simulink model "ZeroForceDrag_SingleJoint"  (R2018b)
settings: Solver=FixedStepDiscrete  StartTime=0.0  StopTime=Inf  FixedStep=0.001  RelTol=1e-3  EnableMultiTasking=on
undefined symbols (not defined in the file): J1, J2, J3, J4, J5, J6, J7, Motor_Current, Motor_Position, Motor_Velocity, Send_GUIdata
libraries: c280xlib x14, simulink x5, idelinklib_common x1
(part 1 of 4)
settings Model: ExtModeTrigDuration=8  Creator=Administrator  LastModifiedBy=Jeason
settings OptimizationCC: DefaultUnderspecifiedDataType=single  EnhancedBackFolding=on  PassReuseOutputArgsAs=Individual arguments  MaxStackSize=512  OptimizeBlockOrder=speed  DifferentSizesBufferReuse=on  OptimizationCustomize=off
settings DebuggingCC: InheritedTsInSrcMsg=none  MultiTaskDSMMsg=none  ParameterTunabilityLossMsg=error
settings HardwareCC: ProdBitPerChar=16  ProdBitPerInt=16  ProdBitPerPointer=32  ProdBitPerSizeT=32  ProdBitPerPtrDiffT=32  ProdLargestAtomicInteger=Integer  ProdLargestAtomicFloat=None  ProdWordSize=16  ProdLongLongMode=on  ProdHWDeviceType=Texas Instruments->C2000
settings SFSimCC: MATLABDynamicMemAlloc=off
settings RTWCC: SystemTargetFile=ert.tlc  HardwareBoard=TI Delfino F2833x  TemplateMakefile=ert_default_tmf  GenerateReport=on  Toolchain=Texas Instruments Code Composer Studio (C2000)  IncludeHyperlinkInReport=on  LaunchReport=on  GenerateTraceInfo=on  GenerateTraceReport=on  GenerateTraceReportSl=on  GenerateTraceReportSf=on  GenerateTraceReportEml=on
settings CodeAppCC: ForceParamTrailComments=on  IgnoreCustomStorageClasses=off  OperatorAnnotations=on  SimulinkDataObjDesc=on  SFDataObjDesc=on  InsertBlockDesc=on
settings ERTTargetCC: CodeReplacementLibrary=TI C28x

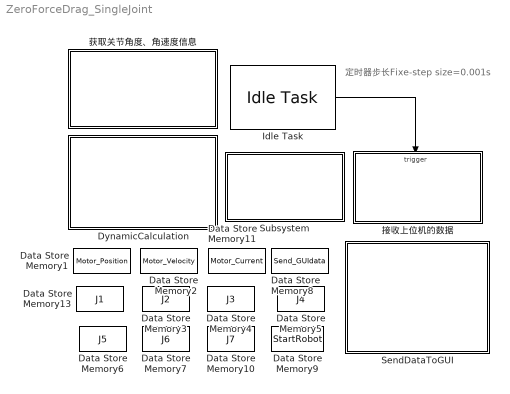
== system ZeroForceDrag_SingleJoint ==
  note: 定时器步长Fixe-step size=0.001s
  Data Store Memory1 : DataStoreMemory  DataStoreName=Motor_Position  ReadBeforeWriteMsg=warning  WriteAfterWriteMsg=warning  WriteAfterReadMsg=warning  InitialValue=[0 0 0 0 0 0]  ShowAdditionalParam=off  OutDataTypeStr=int32
      settings: RTWStateStorageClass=ExportedGlobal
  Data Store Memory10 : DataStoreMemory  DataStoreName=J7  ReadBeforeWriteMsg=warning  WriteAfterWriteMsg=warning  WriteAfterReadMsg=warning  InitialValue=[0 0 0 0 0 0]  ShowAdditionalParam=off  OutDataTypeStr=double
      settings: RTWStateStorageClass=ExportedGlobal
  Data Store Memory11 : DataStoreMemory  DataStoreName=Motor_Current  ReadBeforeWriteMsg=warning  WriteAfterWriteMsg=warning  WriteAfterReadMsg=warning  InitialValue=[0 0 0 0 0 0]  ShowAdditionalParam=off  OutDataTypeStr=int32
      settings: RTWStateStorageClass=ExportedGlobal
  Data Store Memory13 : DataStoreMemory  DataStoreName=J1  ReadBeforeWriteMsg=warning  WriteAfterWriteMsg=warning  WriteAfterReadMsg=warning  InitialValue=[0 0 0 0 0 0]  ShowAdditionalParam=off  OutDataTypeStr=double
      settings: RTWStateStorageClass=ExportedGlobal
  Data Store Memory2 : DataStoreMemory  DataStoreName=Motor_Velocity  ReadBeforeWriteMsg=warning  WriteAfterWriteMsg=warning  WriteAfterReadMsg=warning  InitialValue=[0 0 0 0 0 0]  ShowAdditionalParam=off  OutDataTypeStr=int32
      settings: RTWStateStorageClass=ExportedGlobal
  Data Store Memory3 : DataStoreMemory  DataStoreName=J2  ReadBeforeWriteMsg=warning  WriteAfterWriteMsg=warning  WriteAfterReadMsg=warning  InitialValue=[0 0 0 0 0 0]  ShowAdditionalParam=off  OutDataTypeStr=double
      settings: RTWStateStorageClass=ExportedGlobal
  Data Store Memory4 : DataStoreMemory  DataStoreName=J3  ReadBeforeWriteMsg=warning  WriteAfterWriteMsg=warning  WriteAfterReadMsg=warning  InitialValue=[0 0 0 0 0 0]  ShowAdditionalParam=off  OutDataTypeStr=double
      settings: RTWStateStorageClass=ExportedGlobal
  Data Store Memory5 : DataStoreMemory  DataStoreName=J4  ReadBeforeWriteMsg=warning  WriteAfterWriteMsg=warning  WriteAfterReadMsg=warning  InitialValue=[0 0 0 0 0 0]  ShowAdditionalParam=off  OutDataTypeStr=double
      settings: RTWStateStorageClass=ExportedGlobal
  Data Store Memory6 : DataStoreMemory  DataStoreName=J5  ReadBeforeWriteMsg=warning  WriteAfterWriteMsg=warning  WriteAfterReadMsg=warning  InitialValue=[0 0 0 0 0 0]  ShowAdditionalParam=off  OutDataTypeStr=double
      settings: RTWStateStorageClass=ExportedGlobal
  Data Store Memory7 : DataStoreMemory  DataStoreName=J6  ReadBeforeWriteMsg=warning  WriteAfterWriteMsg=warning  WriteAfterReadMsg=warning  InitialValue=[0 0 0 0 0 0]  ShowAdditionalParam=off  OutDataTypeStr=double
      settings: RTWStateStorageClass=ExportedGlobal
  Data Store Memory8 : DataStoreMemory  DataStoreName=Send_GUIdata  ReadBeforeWriteMsg=warning  WriteAfterWriteMsg=warning  WriteAfterReadMsg=warning  InitialValue=zeros(1,18)  ShowAdditionalParam=off  OutDataTypeStr=double
      settings: RTWStateStorageClass=ExportedGlobal
  Data Store Memory9 : DataStoreMemory  DataStoreName=StartRobot  ReadBeforeWriteMsg=warning  WriteAfterWriteMsg=warning  WriteAfterReadMsg=warning  ShowAdditionalParam=off  OutDataTypeStr=uint16
      settings: RTWStateStorageClass=ExportedGlobal
  DynamicCalculation : Subsystem  Tag=Calculated_Data  Priority=2  TreatAsAtomicUnit=on  RTWFcnName=DynamicsController
      settings: RTWSystemCode=Nonreusable function  RTWFcnNameOpts=User specified  RTWFileNameOpts=Use function name
      mask Display:
      | color('red')
      | disp('六轴机械臂\n单关节零力控制')
  Idle Task : idelinklib_common/Idle Task  tasknumbers=[0]  taskpriorities=100016  taskpreempts=[1]  showinput=off  simPriority=0
  SendDataToGUI : Subsystem  Priority=2  TreatAsAtomicUnit=on
      settings: RTWSystemCode=Nonreusable function
  Subsystem : Subsystem
      mask Display: disp('System\nInitialization');
  接收上位机的数据 : Subsystem  TreatAsAtomicUnit=on
  获取关节角度、角速度信息 : Subsystem  Tag=Get_Data  Priority=0  TreatAsAtomicUnit=on
      settings: RTWSystemCode=Nonreusable function
  wires:
  Idle Task/1 -> 接收上位机的数据/Trigger

== system ZeroForceDrag_SingleJoint/DynamicCalculation ==
  note: 转换为外转子的角度值
  note: 定义全局变量，各变量
      | 为[1x6]的矩阵
  note: 六轴机械臂单关节零力拖动
      | 默认关节2
  note: 在做实验时选择对应的关节电机
  note: 注：必须两人操作，一人扶着机械臂，另外一人负责操作软硬件。以下是简化版的步骤，具体细节以实验指导书为准。
      | 首先打开稳压电源开关给机械臂控制器供电，然后再打开机械臂电源开关,上电2~3s后，打开上位机，点击上位机示教界面的“ 启动 ”按钮，所有电机松开抱闸。
      | 上位机的“ 组号 ”输入 7 ，“ 数据1 ”输入 1 ，点击" 下发数据 "按钮，对应电机切换到力矩模式，然后用手托着机械臂，防止重力原因掉落。
      | 上位机的“ 组号 ”输入对应关节组号，“ 数据1~数据6 ”输入对应的数据，点击" 下发数据 "按钮，输出力矩值给电机。
      | 做完实验后，按下急停按钮，断开机械臂电源，机械臂切换到位置模式，处于锁死状态。（要想让机械臂所有关节回到零位置，需下载PTP程序）。
  Compensate : Subsystem  Priority=1  TreatAsAtomicUnit=on  RTWFcnName=Compensate
      settings: RTWSystemCode=Nonreusable function  RTWFcnNameOpts=User specified  RTWFileNameOpts=Use function name
  Data Store Write3 : DataStoreWrite  DataStoreName=Tau  DataStoreElements=Tau(1)#Tau(2)#Tau(3)#Tau(4)#Tau(5)#Tau(6)
  Demux : Demux  Outputs=6
  DriveMotor : Subsystem  TreatAsAtomicUnit=on  RTWFcnName=DrivrMotor  mask(DriverMotor){Motor1=off, Motor2=on, Motor3=off, Motor4=off, Motor5=off, Motor6=off}
      mask help:
      | 当其中一个Motor勾选时，表示将力矩输出给对应的电机；如果不勾选时，表示对应的电机不工作。
      | 比如：如果做单关节实验时，哪个电机要做实验就勾选对应的电机，其他电机一定要不勾选。
      | 关节1~3为CANB,关节4~6为CANA,驱动邮箱号为7~12。输入量的范围限定在-900~900。
      settings: RTWSystemCode=Nonreusable function  RTWFcnNameOpts=User specified  RTWFileNameOpts=Use function name
      mask Callback Motor1:
      | vssBlk1 = [gcb, '/BottomDriver/Joint1'];
      | choice1 = get_param(gcb,'Motor1');
      | if strcmp(choice1,'off')
      |         set_param(vssBlk1, 'Commented','on');
      |     else
      |         set_param(vssBlk1, 'Commented','off');
      | end
      | clear choice1 vssBlk1;
      mask Callback Motor2:
      | vssBlk2 = [gcb, '/BottomDriver/Joint2'];
      | choice2 = get_param(gcb,'Motor2');
      | if strcmp(choice2,'off')
      |         set_param(vssBlk2, 'Commented','on');
      |     else
      |         set_param(vssBlk2, 'Commented','off');
      | end
      | clear choice2 vssBlk2;
      mask Callback Motor3:
      | vssBlk3 = [gcb, '/BottomDriver/Joint3'];
      | choice3 = get_param(gcb,'Motor3');
      | if strcmp(choice3,'off')
      |         set_param(vssBlk3, 'Commented','on');
      |     else
      |         set_param(vssBlk3, 'Commented','off');
      | end
      | clear choice3 vssBlk3;
      mask Callback Motor4:
      | vssBlk4 = [gcb, '/BottomDriver/Joint4'];
      | choice4 = get_param(gcb,'Motor4');
      | if strcmp(choice4,'off')
      |         set_param(vssBlk4, 'Commented','on');
      |     else
      |         set_param(vssBlk4, 'Commented','off');
      | end
      | clear choice4 vssBlk4;
      mask Callback Motor5:
      | vssBlk5 = [gcb, '/BottomDriver/Joint5'];
      | choice5 = get_param(gcb,'Motor5');
      | if strcmp(choice5,'off')
      |         set_param(vssBlk5, 'Commented','on');
      |     else
      |         set_param(vssBlk5, 'Commented','off');
      | end
      | clear choice5 vssBlk5;
      mask Callback Motor6:
      | vssBlk6 = [gcb, '/BottomDriver/Joint6'];
      | choice6 = get_param(gcb,'Motor6');
      | if strcmp(choice6,'off')
      |         set_param(vssBlk6, 'Commented','on');
      |     else
      |         set_param(vssBlk6, 'Commented','off');
      | end
      | clear choice6 vssBlk6;
      mask Display:
      | disp('DriverMotor');
      | port_label('input', 1, 'Tau1');
      | port_label('input', 2, 'Tau2');
      | port_label('input', 3, 'Tau3');
      | port_label('input', 4, 'Tau4');
      | port_label('input', 5, 'Tau5');
      | port_label('input', 6, 'Tau6');
      | port_label('input', 7, 'Enable');
  Gain : Gain  Gain=180/pi
  GetAngleVelocity : Subsystem  Priority=0  TreatAsAtomicUnit=on  RTWFcnName=GetAngleVelocity
      settings: RTWSystemCode=Nonreusable function  RTWFcnNameOpts=User specified  RTWFileNameOpts=Use function name
  InitAngle : DataStoreRead  DataStoreName=InitAngle
  Tau1~6 : DataStoreRead  DataStoreName=Tau
  dq : DataStoreRead  DataStoreName=dq
  q : DataStoreRead  DataStoreName=q
  上位机监控窗口1~6——参数1 : DataStoreWrite  DataStoreName=Send_GUIdata  DataStoreElements=Send_GUIdata(1:6)
  上位机监控窗口1~6——参数2 : DataStoreWrite  DataStoreName=Send_GUIdata  DataStoreElements=Send_GUIdata(7:12)
  切换到电流模式 的使能信号 : DataStoreRead  DataStoreName=J7  DataStoreElements=J7(1)
  各个关节外转子采集 到的原始角度-初始角度 : DataStoreMemory  DataStoreName=q  ReadBeforeWriteMsg=warning  WriteAfterWriteMsg=warning  WriteAfterReadMsg=warning  InitialValue=zeros(1,6)  ShowAdditionalParam=off  OutDataTypeStr=double
      settings: RTWStateStorageClass=ExportedGlobal
  各个关节外转子采集 到的实际角速度 : DataStoreMemory  DataStoreName=dq  ReadBeforeWriteMsg=warning  WriteAfterWriteMsg=warning  WriteAfterReadMsg=warning  InitialValue=zeros(1,6)  ShowAdditionalParam=off  OutDataTypeStr=double
      settings: RTWStateStorageClass=ExportedGlobal
  各关节角度 : DataStoreWrite  DataStoreName=q
  各关节角速度 : DataStoreWrite  DataStoreName=dq
  给定各关节 初始角度 : DataStoreMemory  DataStoreName=InitAngle  ReadBeforeWriteMsg=warning  WriteAfterWriteMsg=warning  WriteAfterReadMsg=warning  InitialValue=zeros(1,6)  ShowAdditionalParam=off  OutDataTypeStr=double
      settings: RTWStateStorageClass=ExportedGlobal
  给定的各关节 初始角度 : DataStoreWrite  DataStoreName=InitAngle
  驱动各个关节 运动的力矩 : DataStoreMemory  DataStoreName=Tau  ReadBeforeWriteMsg=warning  WriteAfterWriteMsg=warning  WriteAfterReadMsg=warning  InitialValue=zeros(1,6)  ShowAdditionalParam=off  OutDataTypeStr=double
      settings: RTWStateStorageClass=ExportedGlobal
  wires:
  Demux/3 -> DriveMotor/3(Tau3)
  Demux/5 -> DriveMotor/5(Tau5)
  Demux/2 -> DriveMotor/2(Tau2)
  Tau1~6/1 -> 上位机监控窗口1~6——参数2/1, Demux/1
  Demux/4 -> DriveMotor/4(Tau4)
  切换到电流模式 的使能信号/1 -> DriveMotor/7(Enable)
  Demux/1 -> DriveMotor/1(Tau1)
  Demux/6 -> DriveMotor/6(Tau6)
  q/1 -> Gain/1, Compensate/1(q)
  dq/1 -> Compensate/3(dq)
  Compensate/1(Tau1) -> Data Store Write3/1
  Compensate/2(Tau2) -> Data Store Write3/2
  Compensate/3(Tau3) -> Data Store Write3/3
  Compensate/4(Tau4) -> Data Store Write3/4
  Compensate/5(Tau5) -> Data Store Write3/5
  Compensate/6(Tau6) -> Data Store Write3/6
  Gain/1 -> 上位机监控窗口1~6——参数1/1
  GetAngleVelocity/2(InitAngle(rad)) -> 给定的各关节 初始角度/1
  GetAngleVelocity/1(q(rad)) -> 各关节角度/1
  GetAngleVelocity/3(q_dot(rad/s)) -> 各关节角速度/1
  InitAngle/1 -> Compensate/2(InitAngle)

== system ZeroForceDrag_SingleJoint/SendDataToGUI ==
  note: Upper limit=9
  note: 发送数据给上位机
  note: 定时器步长Fixe-step size=0.001s,
      | 每10ms发送一次数据给上位机
  " " : Subsystem
  Constant : Constant  Value=true  OutDataTypeStr=boolean
  Constant1 : Constant  Value=false  OutDataTypeStr=boolean
  Switch : Switch  Criteria=u2 > Threshold
  广播周期 : simulink/Sources/Counter Limited  uplimit=9  tsamp=-1
  wires:
  Switch/1 -> " "/Enable
  广播周期/1 -> Switch/2
  Constant1/1 -> Switch/1
  Constant/1 -> Switch/3

== system ZeroForceDrag_SingleJoint/Subsystem ==
  Model Header : Subsystem  mask(Model Header){ShowInLibBrowser=0}
      mask prompts: ShowInLibBrowser "Simulink:masks:CustCodeMaskParam1_MP"
      settings: CopyFcn=cccopyfcn(gcb)  OpenFcn=ccopenfcn('Model Header')
      mask Help: eval('feval(''rtwprivate'',''rtwhelpview'',''rtw_model_header_block'')');
      mask Display: disp('Model\nHeader');
  Model Source : Subsystem  mask(Model Source){ShowInLibBrowser=0}
      mask prompts: ShowInLibBrowser "Simulink:masks:CustCodeMaskParam1_MP"
      settings: CopyFcn=cccopyfcn(gcb)  OpenFcn=ccopenfcn('Model Source')
      mask Help: eval('feval(''rtwprivate'',''rtwhelpview'',''rtw_model_source_block'')');
      mask Display: disp('Model\nSource');
  System Initialize : Subsystem  mask(System Initialize){ShowInLibBrowser=0}
      mask prompts: ShowInLibBrowser "Simulink:masks:CustCodeMaskParam1_MP"
      settings: CopyFcn=cccopyfcn(gcb)  OpenFcn=ccopenfcn('System Initialize Function')
      mask Help: eval('feval(''rtwprivate'',''rtwhelpview'',''rtw_sys_initialize_block'')');
      mask Display: disp('System\nInitialize');

== system ZeroForceDrag_SingleJoint/接收上位机的数据 ==
  note: 接收上位机数据
  function : TriggerPort  TriggerType=function-call  VariantControl=Variant
  0x0080 : simulink/Logic and Bit Operations/Compare To Constant  relop===  const=hex2dec('0080')  OutDataTypeStr=boolean
  0x88 : simulink/Logic and Bit Operations/Compare To Constant  relop===  const=hex2dec('0088')  OutDataTypeStr=boolean
  Compare To Constant1 : simulink/Logic and Bit Operations/Compare To Constant  relop===  const=hex2dec('0001')  OutDataTypeStr=boolean
  Compare To Constant2 : simulink/Logic and Bit Operations/Compare To Constant  relop===  const=hex2dec('0001')  OutDataTypeStr=boolean
  Data Store Read : DataStoreRead  DataStoreName=PTX
  Data Store Write2 : DataStoreWrite  DataStoreName=StartRobot
  Data Type Conversion : DataTypeConversion  OutDataTypeStr=int16
  Data Type Conversion3 : DataTypeConversion  OutDataTypeStr=double
  Data Type Conversion4 : DataTypeConversion  OutDataTypeStr=uint16
  Demux1 : Demux  Outputs=9
  Logical Operator : Logic  Inputs=4  AllPortsSameDT=off  OutDataTypeStr=boolean
  Mux1 : Mux  Inputs=6
  Subsystem : Subsystem
  Terminator3 : Terminator
  消息使能 : DataStoreMemory  DataStoreName=PTX  ReadBeforeWriteMsg=warning  WriteAfterWriteMsg=warning  WriteAfterReadMsg=warning  InitialValue=true  ShowAdditionalParam=off  OutDataTypeStr=boolean
  获取用户命令 : Subsystem  Priority=1  TreatAsAtomicUnit=on
      settings: RTWSystemCode=Nonreusable function
  wires:
  Compare To Constant2/1 -> Logical Operator/4
  Compare To Constant1/1 -> Logical Operator/3
  Data Store Read/1 -> Logical Operator/2
  Logical Operator/1 -> Data Type Conversion4/1
  0x0080/1 -> Logical Operator/1
  Demux1/4 -> Mux1/2, Compare To Constant2/1
  Demux1/3 -> Mux1/1, Compare To Constant1/1
  Demux1/1 -> 0x0080/1, 0x88/1
  获取用户命令/1(消息) -> Demux1/1
  Demux1/5 -> Mux1/3
  Demux1/6 -> Mux1/4
  Demux1/9 -> Terminator3/1
  Demux1/7 -> Mux1/5
  Demux1/8 -> Mux1/6
  Mux1/1 -> Data Type Conversion/1
  Data Type Conversion/1 -> Data Type Conversion3/1
  Data Type Conversion4/1 -> Data Store Write2/1
  Demux1/2 -> Subsystem/1(组号)
  Data Type Conversion3/1 -> Subsystem/2(数据)
  0x88/1 -> Subsystem/Enable

== system ZeroForceDrag_SingleJoint/获取关节角度、角速度信息 ==
  note: 获取关节电流、 角速度、 角度信息
  CANA_284_24 : Subsystem  Priority=4  TreatAsAtomicUnit=on
      settings: RTWSystemCode=Nonreusable function
      mask Display:
      | color('WHITE')
      | disp('JOINT4\n数据读取')
  CANA_285_25 : Subsystem  Priority=5  TreatAsAtomicUnit=on
      settings: RTWSystemCode=Nonreusable function
      mask Display:
      | color('WHITE')
      | disp('JOINT5\n数据读取')
  CANA_286_26 : Subsystem  Priority=6  TreatAsAtomicUnit=on
      settings: RTWSystemCode=Nonreusable function
      mask Display:
      | color('WHITE')
      | disp('JOINT6\n数据读取')
  CANB_281_21 : Subsystem  Priority=1  TreatAsAtomicUnit=on
      settings: RTWSystemCode=Nonreusable function
      mask Display:
      | color('WHITE')
      | disp('JOINT1\n数据读取')
  CANB_282_22 : Subsystem  Priority=2  TreatAsAtomicUnit=on
      settings: RTWSystemCode=Nonreusable function
      mask Display:
      | color('white')
      | disp('JOINT2\n数据读取')
  CANB_283_23 : Subsystem  Priority=3  TreatAsAtomicUnit=on
      settings: RTWSystemCode=Nonreusable function
      mask Display:
      | color('white')
      | disp('JOINT3\n数据读取')

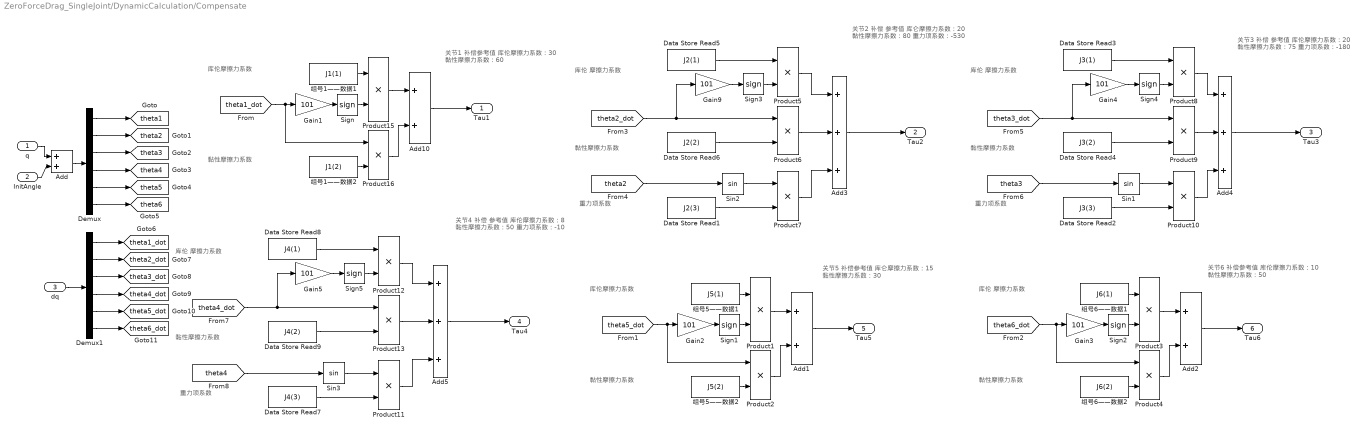
== system ZeroForceDrag_SingleJoint/DynamicCalculation/Compensate ==
  note: 关节1 补偿参考值
      | 库伦摩擦力系数：30
      | 黏性摩擦力系数：60
  note: 关节6 补偿参考值
      | 库伦摩擦力系数：10
      | 黏性摩擦力系数：50
  note: 库伦摩擦力系数
  note: 关节5 补偿参考值
      | 库仑摩擦力系数：15
      | 黏性摩擦力系数：30
  note: 黏性摩擦力系数
  note: 库伦摩擦力系数
  note: 黏性摩擦力系数
  note: 库伦 摩擦力系数
  note: 黏性摩擦力系数
  note: 黏性摩擦力系数
  note: 关节2 补偿 参考值
      | 库仑摩擦力系数：20
      | 黏性摩擦力系数：80
      | 重力项系数：-530
  note: 重力项系数
  note: 库伦 摩擦力系数
  note: 黏性摩擦力系数
  note: 关节3 补偿 参考值
      | 库伦摩擦力系数：20
      | 黏性摩擦力系数：75
      | 重力项系数：-180
  note: 重力项系数
  note: 库伦 摩擦力系数
  note: 黏性摩擦力系数
  note: 关节4 补偿 参考值
      | 库伦摩擦力系数：8
      | 黏性摩擦力系数：50
      | 重力项系数：-10
  note: 重力项系数
  note: 库伦 摩擦力系数
  q : Inport
  InitAngle : Inport  Port=2
  dq : Inport  Port=3
  Add{,1..2,10} (4 alike) : Sum
  Add3 : Sum  Inputs=+++
  Add4 : Sum  Inputs=+++
  Add5 : Sum  Inputs=+++
  Data Store Read1 : DataStoreRead  DataStoreName=J2  DataStoreElements=J2(3)
  Data Store Read2 : DataStoreRead  DataStoreName=J3  DataStoreElements=J3(3)
  Data Store Read3 : DataStoreRead  DataStoreName=J3  DataStoreElements=J3(1)
  Data Store Read4 : DataStoreRead  DataStoreName=J3  DataStoreElements=J3(2)
  Data Store Read5 : DataStoreRead  DataStoreName=J2  DataStoreElements=J2(1)
  Data Store Read6 : DataStoreRead  DataStoreName=J2  DataStoreElements=J2(2)
  Data Store Read7 : DataStoreRead  DataStoreName=J4  DataStoreElements=J4(3)
  Data Store Read8 : DataStoreRead  DataStoreName=J4  DataStoreElements=J4(1)
  Data Store Read9 : DataStoreRead  DataStoreName=J4  DataStoreElements=J4(2)
  Demux : Demux  Outputs=6
  Demux1 : Demux  Outputs=6
  Gain{1..5,9} (6 alike) : Gain  Gain=101
  Product{1,3,5,7..8,10..12,15} (9 alike) : Product
  Product{2,4,6,9,13,16} (6 alike) : Product  OutDataTypeStr=double
  Sign{,1..5} (6 alike) : Signum
  Sin1 : Trigonometry
  Sin2 : Trigonometry
  Sin3 : Trigonometry
  组号1——数据1 : DataStoreRead  DataStoreName=J1  DataStoreElements=J1(1)
  组号1——数据2 : DataStoreRead  DataStoreName=J1  DataStoreElements=J1(2)
  组号5——数据1 : DataStoreRead  DataStoreName=J5  DataStoreElements=J5(1)
  组号5——数据2 : DataStoreRead  DataStoreName=J5  DataStoreElements=J5(2)
  组号6——数据1 : DataStoreRead  DataStoreName=J6  DataStoreElements=J6(1)
  组号6——数据2 : DataStoreRead  DataStoreName=J6  DataStoreElements=J6(2)
  Tau1 : Outport
  Tau2 : Outport  Port=2
  Tau3 : Outport  Port=3
  Tau4 : Outport  Port=4
  Tau5 : Outport  Port=5
  Tau6 : Outport  Port=6
  tag scope: theta1=global, theta1_dot=global, theta2=global, theta2_dot=global, theta3=global, theta3_dot=global, theta4=global, theta4_dot=global, theta5=global, theta5_dot=global, theta6=global, theta6_dot=global
  wires:
  [theta1_dot] -> Product16/1, Gain1/1
  Sign/1 -> Product15/2
  Product16/1 -> Add10/2
  Product15/1 -> Add10/1
  Gain1/1 -> Sign/1
  组号1——数据1/1 -> Product15/1
  Add10/1 -> Tau1/1
  组号1——数据2/1 -> Product16/2
  组号5——数据2/1 -> Product2/2
  Add1/1 -> Tau5/1
  组号5——数据1/1 -> Product1/1
  Gain2/1 -> Sign1/1
  Product1/1 -> Add1/1
  Product2/1 -> Add1/2
  Sign1/1 -> Product1/2
  [theta5_dot] -> Gain2/1, Product2/1
  [theta6_dot] -> Product4/1, Gain3/1
  Sign2/1 -> Product3/2
  Product4/1 -> Add2/2
  Product3/1 -> Add2/1
  Gain3/1 -> Sign2/1
  组号6——数据1/1 -> Product3/1
  Add2/1 -> Tau6/1
  组号6——数据2/1 -> Product4/2
  Gain9/1 -> Sign3/1
  Data Store Read5/1 -> Product5/1
  Product7/1 -> Add3/3
  Sin2/1 -> Product7/1
  Product5/1 -> Add3/1
  Product6/1 -> Add3/2
  [theta2] -> Sin2/1
  Data Store Read6/1 -> Product6/2
  Data Store Read1/1 -> Product7/2
  [theta2_dot] -> Gain9/1, Product6/1
  Sign3/1 -> Product5/2
  Add3/1 -> Tau2/1
  dq/1 -> Demux1/1
  Demux/1 -> [theta1]
  Demux/2 -> [theta2]
  Demux/3 -> [theta3]
  Demux/4 -> [theta4]
  Demux/5 -> [theta5]
  Demux/6 -> [theta6]
  Demux1/1 -> [theta1_dot]
  Demux1/2 -> [theta2_dot]
  Demux1/3 -> [theta3_dot]
  Demux1/4 -> [theta4_dot]
  Demux1/5 -> [theta5_dot]
  Demux1/6 -> [theta6_dot]
  Add4/1 -> Tau3/1
  Sign4/1 -> Product8/2
  [theta3_dot] -> Product9/1, Gain4/1
  Data Store Read2/1 -> Product10/2
  Data Store Read4/1 -> Product9/2
  [theta3] -> Sin1/1
  Product9/1 -> Add4/2
  Product8/1 -> Add4/1
  Sin1/1 -> Product10/1
  Product10/1 -> Add4/3
  Data Store Read3/1 -> Product8/1
  Gain4/1 -> Sign4/1
  Gain5/1 -> Sign5/1
  Data Store Read8/1 -> Product12/1
  Product11/1 -> Add5/3
  Sin3/1 -> Product11/1
  Product12/1 -> Add5/1
  Product13/1 -> Add5/2
  [theta4] -> Sin3/1
  Data Store Read9/1 -> Product13/2
  Data Store Read7/1 -> Product11/2
  [theta4_dot] -> Gain5/1, Product13/1
  Sign5/1 -> Product12/2
  Add5/1 -> Tau4/1
  InitAngle/1 -> Add/2
  q/1 -> Add/1
  Add/1 -> Demux/1

== system ZeroForceDrag_SingleJoint/DynamicCalculation/DriveMotor ==
  Tau1 : Inport
  Tau2 : Inport  Port=2
  Tau3 : Inport  Port=3
  Tau4 : Inport  Port=4
  Tau5 : Inport  Port=5
  Tau6 : Inport  Port=6
  Enable : Inport  Port=7
  BottomDriver : Subsystem
  Data Store Memory1 : DataStoreMemory  DataStoreName=TXD  ReadBeforeWriteMsg=warning  WriteAfterWriteMsg=warning  WriteAfterReadMsg=warning  InitialValue=[0]  ShowAdditionalParam=off  OutDataTypeStr=uint8
      settings: RTWStateStorageClass=ExportedGlobal
  Data Store Read4 : DataStoreRead  DataStoreName=TXD
  Saturation{1..6} (6 alike) : Saturate  UpperLimit=900  LowerLimit=-900
  驱动器指令 : Subsystem  TreatAsAtomicUnit=on
      settings: RTWSystemCode=Nonreusable function
  wires:
  Data Store Read4/1 -> BottomDriver/Enable
  驱动器指令/4(MSG4) -> BottomDriver/4(JOINT4)
  驱动器指令/3(MSG3) -> BottomDriver/3(JOINT3)
  驱动器指令/1(MSG1) -> BottomDriver/1(JOINT1)
  驱动器指令/2(MSG2) -> BottomDriver/2(JOINT2)
  Enable/1 -> 驱动器指令/7(Enable)
  驱动器指令/5(MSG5) -> BottomDriver/5(JOINT5)
  Saturation2/1 -> 驱动器指令/1(Current1)
  Saturation1/1 -> 驱动器指令/2(Current2)
  Saturation3/1 -> 驱动器指令/3(Current3)
  Saturation4/1 -> 驱动器指令/4(Current4)
  Saturation5/1 -> 驱动器指令/5(Current5)
  Tau1/1 -> Saturation2/1
  Tau2/1 -> Saturation1/1
  Tau3/1 -> Saturation3/1
  Tau4/1 -> Saturation4/1
  Tau5/1 -> Saturation5/1
  驱动器指令/6(MSG6) -> BottomDriver/6(JOINT6)
  Tau6/1 -> Saturation6/1
  Saturation6/1 -> 驱动器指令/6(Current6)

== system ZeroForceDrag_SingleJoint/DynamicCalculation/GetAngleVelocity ==
  GetAngle1 : Subsystem  TreatAsAtomicUnit=on  mask(获取电机外转子角度(rad)){JJoint=1, InitAngle=0}
      mask prompts: JJoint "选择关节电机"; InitAngle "给定初始角度(deg)"
      mask help:
      | 给定初始角度：假设在数学建模时，设定连杆在水平位置为0°，而机械臂每个关节在出厂时都设定在竖直位置为0°，那么这里就需要给定一个偏置值90°/-90°，默认设为0。
      | 注：关节3因为结构原因实际获取到的角度的正负和标签贴的方向相反。
      | Angle(rad)=电机外转子的实际角度值-给定的初始角度值
      | InitAngle(rad)=给定的初始角度值
      mask TypeOptions JJoint: 1 | 2 | 3 | 4 | 5 | 6
      mask Display:
      | choice1 = get_param(gcb,'JJoint');
      | color('black');
      | switch choice1
      |     case '1'
      |         disp('获取关节1电机\n外转子角度(rad)');
      |     case '2'
      |         disp('获取关节2电机\n外转子角度(rad)');
      |     case '3'
      |         disp('获取关节3电机\n外转子角度(rad)');
      |     case '4'
      |         disp('获取关节4电机\n外转子角度(rad)');
      |     case '5'
      |         disp('获取关节5电机\n外转子角度(rad)');
      |     case '6'
      |         disp('获取关节6电机\n外转子角度(rad)');
      | end
      | color('black');
      | port_label('output', 1, 'Angle');
      | port_label('output', 2, 'InitAngle');
      | clear choice1;
  GetAngle2 : Subsystem  TreatAsAtomicUnit=on  mask(获取电机外转子角度(rad)){JJoint=2, InitAngle=0}
      mask prompts: JJoint "选择关节电机"; InitAngle "给定初始角度(deg)"
      mask help:
      | 给定初始角度：假设在数学建模时，设定连杆在水平位置为0°，而机械臂每个关节在出厂时都设定在竖直位置为0°，那么这里就需要给定一个偏置值90°/-90°，默认设为0。
      | 注：关节3因为结构原因实际获取到的角度的正负和标签贴的方向相反。
      | Angle(rad)=电机外转子的实际角度值-给定的初始角度值
      | InitAngle(rad)=给定的初始角度值
      mask TypeOptions JJoint: 1 | 2 | 3 | 4 | 5 | 6
      mask Display:
      | choice1 = get_param(gcb,'JJoint');
      | color('black');
      | switch choice1
      |     case '1'
      |         disp('获取关节1电机\n外转子角度(rad)');
      |     case '2'
      |         disp('获取关节2电机\n外转子角度(rad)');
      |     case '3'
      |         disp('获取关节3电机\n外转子角度(rad)');
      |     case '4'
      |         disp('获取关节4电机\n外转子角度(rad)');
      |     case '5'
      |         disp('获取关节5电机\n外转子角度(rad)');
      |     case '6'
      |         disp('获取关节6电机\n外转子角度(rad)');
      | end
      | color('black');
      | port_label('output', 1, 'Angle');
      | port_label('output', 2, 'InitAngle');
      | clear choice1;
  GetAngle3 : Subsystem  TreatAsAtomicUnit=on  mask(获取电机外转子角度(rad)){JJoint=3, InitAngle=0}
      mask prompts: JJoint "选择关节电机"; InitAngle "给定初始角度(deg)"
      mask help:
      | 给定初始角度：假设在数学建模时，设定连杆在水平位置为0°，而机械臂每个关节在出厂时都设定在竖直位置为0°，那么这里就需要给定一个偏置值90°/-90°，默认设为0。
      | 注：关节3因为结构原因实际获取到的角度的正负和标签贴的方向相反。
      | Angle(rad)=电机外转子的实际角度值-给定的初始角度值
      | InitAngle(rad)=给定的初始角度值
      mask TypeOptions JJoint: 1 | 2 | 3 | 4 | 5 | 6
      mask Display:
      | choice1 = get_param(gcb,'JJoint');
      | color('black');
      | switch choice1
      |     case '1'
      |         disp('获取关节1电机\n外转子角度(rad)');
      |     case '2'
      |         disp('获取关节2电机\n外转子角度(rad)');
      |     case '3'
      |         disp('获取关节3电机\n外转子角度(rad)');
      |     case '4'
      |         disp('获取关节4电机\n外转子角度(rad)');
      |     case '5'
      |         disp('获取关节5电机\n外转子角度(rad)');
      |     case '6'
      |         disp('获取关节6电机\n外转子角度(rad)');
      | end
      | color('black');
      | port_label('output', 1, 'Angle');
      | port_label('output', 2, 'InitAngle');
      | clear choice1;
  GetAngle4 : Subsystem  TreatAsAtomicUnit=on  mask(获取电机外转子角度(rad)){JJoint=4, InitAngle=0}
      mask prompts: JJoint "选择关节电机"; InitAngle "给定初始角度(deg)"
      mask help:
      | 给定初始角度：假设在数学建模时，设定连杆在水平位置为0°，而机械臂每个关节在出厂时都设定在竖直位置为0°，那么这里就需要给定一个偏置值90°/-90°，默认设为0。
      | 注：关节3因为结构原因实际获取到的角度的正负和标签贴的方向相反。
      | Angle(rad)=电机外转子的实际角度值-给定的初始角度值
      | InitAngle(rad)=给定的初始角度值
      mask TypeOptions JJoint: 1 | 2 | 3 | 4 | 5 | 6
      mask Display:
      | choice1 = get_param(gcb,'JJoint');
      | color('black');
      | switch choice1
      |     case '1'
      |         disp('获取关节1电机\n外转子角度(rad)');
      |     case '2'
      |         disp('获取关节2电机\n外转子角度(rad)');
      |     case '3'
      |         disp('获取关节3电机\n外转子角度(rad)');
      |     case '4'
      |         disp('获取关节4电机\n外转子角度(rad)');
      |     case '5'
      |         disp('获取关节5电机\n外转子角度(rad)');
      |     case '6'
      |         disp('获取关节6电机\n外转子角度(rad)');
      | end
      | color('black');
      | port_label('output', 1, 'Angle');
      | port_label('output', 2, 'InitAngle');
      | clear choice1;
  GetAngle5 : Subsystem  TreatAsAtomicUnit=on  mask(获取电机外转子角度(rad)){JJoint=5, InitAngle=0}
      mask prompts: JJoint "选择关节电机"; InitAngle "给定初始角度(deg)"
      mask help:
      | 给定初始角度：假设在数学建模时，设定连杆在水平位置为0°，而机械臂每个关节在出厂时都设定在竖直位置为0°，那么这里就需要给定一个偏置值90°/-90°，默认设为0。
      | 注：关节3因为结构原因实际获取到的角度的正负和标签贴的方向相反。
      | Angle(rad)=电机外转子的实际角度值-给定的初始角度值
      | InitAngle(rad)=给定的初始角度值
      mask TypeOptions JJoint: 1 | 2 | 3 | 4 | 5 | 6
      mask Display:
      | choice1 = get_param(gcb,'JJoint');
      | color('black');
      | switch choice1
      |     case '1'
      |         disp('获取关节1电机\n外转子角度(rad)');
      |     case '2'
      |         disp('获取关节2电机\n外转子角度(rad)');
      |     case '3'
      |         disp('获取关节3电机\n外转子角度(rad)');
      |     case '4'
      |         disp('获取关节4电机\n外转子角度(rad)');
      |     case '5'
      |         disp('获取关节5电机\n外转子角度(rad)');
      |     case '6'
      |         disp('获取关节6电机\n外转子角度(rad)');
      | end
      | color('black');
      | port_label('output', 1, 'Angle');
      | port_label('output', 2, 'InitAngle');
      | clear choice1;
  GetAngle6 : Subsystem  TreatAsAtomicUnit=on  mask(获取电机外转子角度(rad)){JJoint=6, InitAngle=0}
      mask prompts: JJoint "选择关节电机"; InitAngle "给定初始角度(deg)"
      mask help:
      | 给定初始角度：假设在数学建模时，设定连杆在水平位置为0°，而机械臂每个关节在出厂时都设定在竖直位置为0°，那么这里就需要给定一个偏置值90°/-90°，默认设为0。
      | 注：关节3因为结构原因实际获取到的角度的正负和标签贴的方向相反。
      | Angle(rad)=电机外转子的实际角度值-给定的初始角度值
      | InitAngle(rad)=给定的初始角度值
      mask TypeOptions JJoint: 1 | 2 | 3 | 4 | 5 | 6
      mask Display:
      | choice1 = get_param(gcb,'JJoint');
      | color('black');
      | switch choice1
      |     case '1'
      |         disp('获取关节1电机\n外转子角度(rad)');
      |     case '2'
      |         disp('获取关节2电机\n外转子角度(rad)');
      |     case '3'
      |         disp('获取关节3电机\n外转子角度(rad)');
      |     case '4'
      |         disp('获取关节4电机\n外转子角度(rad)');
      |     case '5'
      |         disp('获取关节5电机\n外转子角度(rad)');
      |     case '6'
      |         disp('获取关节6电机\n外转子角度(rad)');
      | end
      | color('black');
      | port_label('output', 1, 'Angle');
      | port_label('output', 2, 'InitAngle');
      | clear choice1;
  GetAngleSpeed : Subsystem  Priority=2  TreatAsAtomicUnit=on  mask{JJoint=1}
      mask prompts: JJoint "选择关节电机"
      mask help: 读取电机角速度(rad/s)
      mask TypeOptions JJoint: 1 | 2 | 3 | 4 | 5 | 6
      mask Display:
      | choice1 = get_param(gcb,'JJoint');
      | color('black');
      | switch choice1
      |     case '1'
      |         disp('获取关节1电机\n外转子角速度(rad/s)');
      |     case '2'
      |         disp('获取关节2电机\n外转子角速度(rad/s)');
      |     case '3'
      |         disp('获取关节3电机\n外转子角速度(rad/s)');
      |     case '4'
      |         disp('获取关节4电机\n外转子角速度(rad/s)');
      |     case '5'
      |         disp('获取关节5电机\n外转子角速度(rad/s)');
      |     case '6'
      |         disp('获取关节6电机\n外转子角速度(rad/s)');
      | end
      | color('black');
      | port_label('output', 1, 'Velocity');
      | clear choice1;
  GetAngleSpeed1 : Subsystem  Priority=2  TreatAsAtomicUnit=on  mask{JJoint=2}
      mask prompts: JJoint "选择关节电机"
      mask help: 读取电机角速度(rad/s)
      mask TypeOptions JJoint: 1 | 2 | 3 | 4 | 5 | 6
      mask Display:
      | choice1 = get_param(gcb,'JJoint');
      | color('black');
      | switch choice1
      |     case '1'
      |         disp('获取关节1电机\n外转子角速度(rad/s)');
      |     case '2'
      |         disp('获取关节2电机\n外转子角速度(rad/s)');
      |     case '3'
      |         disp('获取关节3电机\n外转子角速度(rad/s)');
      |     case '4'
      |         disp('获取关节4电机\n外转子角速度(rad/s)');
      |     case '5'
      |         disp('获取关节5电机\n外转子角速度(rad/s)');
      |     case '6'
      |         disp('获取关节6电机\n外转子角速度(rad/s)');
      | end
      | color('black');
      | port_label('output', 1, 'Velocity');
      | clear choice1;
  GetAngleSpeed2 : Subsystem  Priority=2  TreatAsAtomicUnit=on  mask{JJoint=3}
      mask prompts: JJoint "选择关节电机"
      mask help: 读取电机角速度(rad/s)
      mask TypeOptions JJoint: 1 | 2 | 3 | 4 | 5 | 6
      mask Display:
      | choice1 = get_param(gcb,'JJoint');
      | color('black');
      | switch choice1
      |     case '1'
      |         disp('获取关节1电机\n外转子角速度(rad/s)');
      |     case '2'
      |         disp('获取关节2电机\n外转子角速度(rad/s)');
      |     case '3'
      |         disp('获取关节3电机\n外转子角速度(rad/s)');
      |     case '4'
      |         disp('获取关节4电机\n外转子角速度(rad/s)');
      |     case '5'
      |         disp('获取关节5电机\n外转子角速度(rad/s)');
      |     case '6'
      |         disp('获取关节6电机\n外转子角速度(rad/s)');
      | end
      | color('black');
      | port_label('output', 1, 'Velocity');
      | clear choice1;
  GetAngleSpeed3 : Subsystem  Priority=2  TreatAsAtomicUnit=on  mask{JJoint=4}
      mask prompts: JJoint "选择关节电机"
      mask help: 读取电机角速度(rad/s)
      mask TypeOptions JJoint: 1 | 2 | 3 | 4 | 5 | 6
      mask Display:
      | choice1 = get_param(gcb,'JJoint');
      | color('black');
      | switch choice1
      |     case '1'
      |         disp('获取关节1电机\n外转子角速度(rad/s)');
      |     case '2'
      |         disp('获取关节2电机\n外转子角速度(rad/s)');
      |     case '3'
      |         disp('获取关节3电机\n外转子角速度(rad/s)');
      |     case '4'
      |         disp('获取关节4电机\n外转子角速度(rad/s)');
      |     case '5'
      |         disp('获取关节5电机\n外转子角速度(rad/s)');
      |     case '6'
      |         disp('获取关节6电机\n外转子角速度(rad/s)');
      | end
      | color('black');
      | port_label('output', 1, 'Velocity');
      | clear choice1;
  GetAngleSpeed4 : Subsystem  Priority=2  TreatAsAtomicUnit=on  mask{JJoint=5}
      mask prompts: JJoint "选择关节电机"
      mask help: 读取电机角速度(rad/s)
      mask TypeOptions JJoint: 1 | 2 | 3 | 4 | 5 | 6
      mask Display:
      | choice1 = get_param(gcb,'JJoint');
      | color('black');
      | switch choice1
      |     case '1'
      |         disp('获取关节1电机\n外转子角速度(rad/s)');
      |     case '2'
      |         disp('获取关节2电机\n外转子角速度(rad/s)');
      |     case '3'
      |         disp('获取关节3电机\n外转子角速度(rad/s)');
      |     case '4'
      |         disp('获取关节4电机\n外转子角速度(rad/s)');
      |     case '5'
      |         disp('获取关节5电机\n外转子角速度(rad/s)');
      |     case '6'
      |         disp('获取关节6电机\n外转子角速度(rad/s)');
      | end
      | color('black');
      | port_label('output', 1, 'Velocity');
      | clear choice1;
  GetAngleSpeed5 : Subsystem  Priority=2  TreatAsAtomicUnit=on  mask{JJoint=6}
      mask prompts: JJoint "选择关节电机"
      mask help: 读取电机角速度(rad/s)
      mask TypeOptions JJoint: 1 | 2 | 3 | 4 | 5 | 6
      mask Display:
      | choice1 = get_param(gcb,'JJoint');
      | color('black');
      | switch choice1
      |     case '1'
      |         disp('获取关节1电机\n外转子角速度(rad/s)');
      |     case '2'
      |         disp('获取关节2电机\n外转子角速度(rad/s)');
      |     case '3'
      |         disp('获取关节3电机\n外转子角速度(rad/s)');
      |     case '4'
      |         disp('获取关节4电机\n外转子角速度(rad/s)');
      |     case '5'
      |         disp('获取关节5电机\n外转子角速度(rad/s)');
      |     case '6'
      |         disp('获取关节6电机\n外转子角速度(rad/s)');
      | end
      | color('black');
      | port_label('output', 1, 'Velocity');
      | clear choice1;
  Mux : Mux  Inputs=6
  Mux1 : Mux  Inputs=6
  Mux2 : Mux  Inputs=6
  q(rad) : Outport
  InitAngle(rad) : Outport  Port=2
  q_dot(rad/s) : Outport  Port=3
  wires:
  GetAngle4/1(Angle) -> Mux/4
  GetAngle3/1(Angle) -> Mux/3
  GetAngle5/1(Angle) -> Mux/5
  GetAngle1/1(Angle) -> Mux/1
  GetAngle2/1(Angle) -> Mux/2
  GetAngle6/1(Angle) -> Mux/6
  Mux/1 -> q(rad)/1
  GetAngleSpeed/1(Velcity) -> Mux1/1
  GetAngleSpeed1/1(Velcity) -> Mux1/2
  GetAngleSpeed2/1(Velcity) -> Mux1/3
  GetAngleSpeed3/1(Velcity) -> Mux1/4
  GetAngleSpeed4/1(Velcity) -> Mux1/5
  GetAngleSpeed5/1(Velcity) -> Mux1/6
  Mux1/1 -> q_dot(rad/s)/1
  GetAngle1/2(InitAngle) -> Mux2/1
  GetAngle2/2(InitAngle) -> Mux2/2
  GetAngle3/2(InitAngle) -> Mux2/3
  GetAngle4/2(InitAngle) -> Mux2/4
  GetAngle5/2(InitAngle) -> Mux2/5
  GetAngle6/2(InitAngle) -> Mux2/6
  Mux2/1 -> InitAngle(rad)/1

== system ZeroForceDrag_SingleJoint/SendDataToGUI/  ==
  Enable : EnablePort
  Constant1 : Constant  Value=hex2dec('5a')  OutDataTypeStr=uint16
  Data Store Read4 : DataStoreRead  DataStoreName=Send_GUIdata
  Data Type Conversion12 : DataTypeConversion  OutDataTypeStr=uint16
  Demux : Demux  Outputs=18
  Mux : Mux  Inputs=20
  SCI Transmit : c280xlib/SCI Transmit  sciModule=A  dataHead=''  dataTail=''  postInterrupt=off  numFifo=1
      settings: SourceProductName=Embedded Coder Support Package for Texas Instruments C2000 Processors
  校验码填充 : Sum  Inputs=+++++++++++++++++++  AccumDataTypeStr=uint16
  wires:
  Demux/1 -> Mux/2, 校验码填充/2
  Mux/1 -> SCI Transmit/1
  Demux/3 -> 校验码填充/4, Mux/4
  Demux/14 -> 校验码填充/15, Mux/15
  Demux/9 -> 校验码填充/10, Mux/10
  Demux/5 -> Mux/6, 校验码填充/6
  Demux/2 -> 校验码填充/3, Mux/3
  Data Store Read4/1 -> Data Type Conversion12/1
  Demux/13 -> 校验码填充/14, Mux/14
  Demux/6 -> Mux/7, 校验码填充/7
  Demux/8 -> 校验码填充/9, Mux/9
  Demux/10 -> 校验码填充/11, Mux/11
  Demux/4 -> 校验码填充/5, Mux/5
  Demux/7 -> 校验码填充/8, Mux/8
  Demux/15 -> 校验码填充/16, Mux/16
  Demux/11 -> 校验码填充/12, Mux/12
  Demux/18 -> 校验码填充/19, Mux/19
  Demux/16 -> 校验码填充/17, Mux/17
  Constant1/1 -> 校验码填充/1, Mux/1
  Demux/17 -> 校验码填充/18, Mux/18
  校验码填充/1 -> Mux/20
  Demux/12 -> 校验码填充/13, Mux/13
  Data Type Conversion12/1 -> Demux/1

== system ZeroForceDrag_SingleJoint/Subsystem/Model Header ==

== system ZeroForceDrag_SingleJoint/Subsystem/Model Source ==

== system ZeroForceDrag_SingleJoint/Subsystem/System Initialize ==

== system ZeroForceDrag_SingleJoint/接收上位机的数据/Subsystem ==
  组号 : Inport
  数据 : Inport  Port=2
  Enable : EnablePort
  Joint1 : Subsystem  TreatAsAtomicUnit=on
  Joint2 : Subsystem  TreatAsAtomicUnit=on
  Joint3 : Subsystem  TreatAsAtomicUnit=on
  Joint4 : Subsystem  TreatAsAtomicUnit=on
  Joint5 : Subsystem  TreatAsAtomicUnit=on
  Joint6 : Subsystem  TreatAsAtomicUnit=on
  Joint7 : Subsystem  TreatAsAtomicUnit=on
  Switch Case : SwitchCase  CaseConditions={1 2 3 4 5 6 7}  ShowDefaultCase=off
  wires:
  数据/1 -> Joint7/1(Joint7), Joint5/1(Joint5), Joint4/1(Joint4), Joint3/1(Joint3), Joint2/1(Joint2), Joint1/1(Joint1), Joint6/1(Joint6)
  Switch Case/5 -> Joint5/Action
  Switch Case/6 -> Joint6/Action
  Switch Case/2 -> Joint2/Action
  Switch Case/1 -> Joint1/Action
  Switch Case/3 -> Joint3/Action
  Switch Case/4 -> Joint4/Action
  组号/1 -> Switch Case/1
  Switch Case/7 -> Joint7/Action

== system ZeroForceDrag_SingleJoint/接收上位机的数据/获取用户命令 ==
  " " : c280xlib/SCI Receive  sciModule=A  dataHead=''  dataTail=''  dataType=uint16  dataDim=9  initValue=0  errOption=Output the last received value  errValue=0  sampleTime=-1  outputStatus=on  postInterrupt=off  numFifo=1
      settings: SourceProductName=Embedded Coder Support Package for Texas Instruments C2000 Processors  SourceProductBaseCode=TIC2000
  Constant : Constant  Value=false  OutDataTypeStr=boolean
  Constant1 : Constant  Value=true  OutDataTypeStr=boolean
  Data Store Write1 : DataStoreWrite  DataStoreName=PTX
  Logical Operator : Logic  AllPortsSameDT=off  OutDataTypeStr=boolean
  Switch : Switch  Criteria=u2 > Threshold
  消息校验 : Subsystem
  消息 : Outport
  wires:
  消息校验/2(使能) -> Logical Operator/1
  Switch/1 -> Logical Operator/2
  Constant1/1 -> Switch/3
  " "/2 -> Switch/2
  消息校验/1(消息) -> 消息/1
  " "/1 -> 消息校验/1(数据)
  Logical Operator/1 -> Data Store Write1/1
  Constant/1 -> Switch/1

== system ZeroForceDrag_SingleJoint/获取关节角度、角速度信息/CANA_284_24 ==
  note: 控制器接收ID:0x280+“ID”
  Subsystem1 : Subsystem
  eCAN Receive1 : c280xlib/eCAN Receive  chipFamily=C280x  useModule=eCAN_A  mailboxNo=24  messageID=hex2dec('284')  messageType=Standard (11-bit identifier)  sampleTime=-1  dataType=uint8  initValue=0  outputMessageLength=off  outputMessageTimeStamp=off  postInterrupt=off  interruptLine=0
      settings: SourceProductName=Embedded Coder Support Package for Texas Instruments C2000 Processors  SourceProductBaseCode=TIC2000
  wires:
  eCAN Receive1/2 -> Subsystem1/1(In1)
  eCAN Receive1/1 -> Subsystem1/Trigger

== system ZeroForceDrag_SingleJoint/获取关节角度、角速度信息/CANA_285_25 ==
  note: 控制器接收ID:0x280+“ID”
  Subsystem : Subsystem
  eCAN Receive : c280xlib/eCAN Receive  chipFamily=C280x  useModule=eCAN_A  mailboxNo=25  messageID=hex2dec('285')  messageType=Standard (11-bit identifier)  sampleTime=-1  dataType=uint8  initValue=0  outputMessageLength=off  outputMessageTimeStamp=off  postInterrupt=off  interruptLine=0
      settings: SourceProductName=Embedded Coder Support Package for Texas Instruments C2000 Processors  SourceProductBaseCode=TIC2000
  wires:
  eCAN Receive/2 -> Subsystem/1(In1)
  eCAN Receive/1 -> Subsystem/Trigger

== system ZeroForceDrag_SingleJoint/获取关节角度、角速度信息/CANA_286_26 ==
  note: 控制器接收ID:0x280+“ID”
  Subsystem : Subsystem
  eCAN Receive : c280xlib/eCAN Receive  chipFamily=C280x  useModule=eCAN_A  mailboxNo=26  messageID=hex2dec('286')  messageType=Standard (11-bit identifier)  sampleTime=-1  dataType=uint8  initValue=0  outputMessageLength=off  outputMessageTimeStamp=off  postInterrupt=off  interruptLine=0
      settings: SourceProductName=Embedded Coder Support Package for Texas Instruments C2000 Processors  SourceProductBaseCode=TIC2000
  wires:
  eCAN Receive/2 -> Subsystem/1(In1)
  eCAN Receive/1 -> Subsystem/Trigger

== system ZeroForceDrag_SingleJoint/获取关节角度、角速度信息/CANB_281_21 ==
  note: 控制器接收ID:0x280+“ID”
  Subsystem : Subsystem
  eCAN Receive : c280xlib/eCAN Receive  chipFamily=C280x  useModule=eCAN_B  mailboxNo=21  messageID=hex2dec('281')  messageType=Standard (11-bit identifier)  sampleTime=-1  dataType=uint8  initValue=0  outputMessageLength=off  outputMessageTimeStamp=off  postInterrupt=off  interruptLine=0
      settings: SourceProductName=Embedded Coder Support Package for Texas Instruments C2000 Processors  SourceProductBaseCode=TIC2000
  wires:
  eCAN Receive/2 -> Subsystem/1(In1)
  eCAN Receive/1 -> Subsystem/Trigger

== system ZeroForceDrag_SingleJoint/获取关节角度、角速度信息/CANB_282_22 ==
  note: 控制器接收ID:0x280+“ID”
  Subsystem : Subsystem
  eCAN Receive : c280xlib/eCAN Receive  chipFamily=C280x  useModule=eCAN_B  mailboxNo=22  messageID=hex2dec('282')  messageType=Standard (11-bit identifier)  sampleTime=-1  dataType=uint8  initValue=0  outputMessageLength=off  outputMessageTimeStamp=off  postInterrupt=off  interruptLine=0
      settings: SourceProductName=Embedded Coder Support Package for Texas Instruments C2000 Processors  SourceProductBaseCode=TIC2000
  wires:
  eCAN Receive/2 -> Subsystem/1(In1)
  eCAN Receive/1 -> Subsystem/Trigger

== system ZeroForceDrag_SingleJoint/获取关节角度、角速度信息/CANB_283_23 ==
  note: 控制器接收ID:0x280+“ID”
  Subsystem : Subsystem
  eCAN Receive : c280xlib/eCAN Receive  chipFamily=C280x  useModule=eCAN_B  mailboxNo=23  messageID=hex2dec('283')  messageType=Standard (11-bit identifier)  sampleTime=-1  dataType=uint8  initValue=0  outputMessageLength=off  outputMessageTimeStamp=off  postInterrupt=off  interruptLine=0
      settings: SourceProductName=Embedded Coder Support Package for Texas Instruments C2000 Processors  SourceProductBaseCode=TIC2000
  wires:
  eCAN Receive/2 -> Subsystem/1(In1)
  eCAN Receive/1 -> Subsystem/Trigger

== system ZeroForceDrag_SingleJoint/DynamicCalculation/DriveMotor/BottomDriver ==
  JOINT1 : Inport
  JOINT2 : Inport  Port=2
  JOINT3 : Inport  Port=3
  JOINT4 : Inport  Port=4
  JOINT5 : Inport  Port=5
  JOINT6 : Inport  Port=6
  Enable : EnablePort
  Constant : Constant  Value=0  OutDataTypeStr=uint8
  Data Store Write : DataStoreWrite  DataStoreName=TXD
  Joint1 : Subsystem  Priority=1  Commented=on
  Joint2 : Subsystem  Priority=2
  Joint3 : Subsystem  Priority=3  Commented=on
  Joint4 : Subsystem  Priority=4  Commented=on
  Joint5 : Subsystem  Priority=5  Commented=on
  Joint6 : Subsystem  Priority=6  Commented=on
  wires:
  JOINT3/1 -> Joint3/1(In1)
  JOINT5/1 -> Joint5/1(In1)
  JOINT2/1 -> Joint2/1(In1)
  JOINT4/1 -> Joint4/1(In1)
  JOINT6/1 -> Joint6/1(In1)
  JOINT1/1 -> Joint1/1(In6)
  Constant/1 -> Data Store Write/1

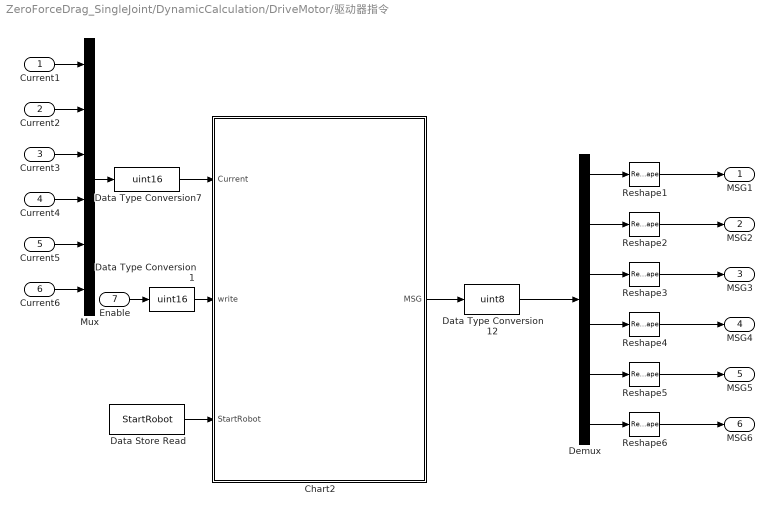
== system ZeroForceDrag_SingleJoint/DynamicCalculation/DriveMotor/驱动器指令 ==
  Current1 : Inport
  Current2 : Inport  Port=2
  Current3 : Inport  Port=3
  Current4 : Inport  Port=4
  Current5 : Inport  Port=5
  Current6 : Inport  Port=6
  Enable : Inport  Port=7
  Chart2 : Stateflow chart  TreatAsAtomicUnit=on
  Data Store Read : DataStoreRead  DataStoreName=StartRobot
  Data Type Conversion1 : DataTypeConversion  OutDataTypeStr=uint16
  Data Type Conversion12 : DataTypeConversion  OutDataTypeStr=uint8
  Data Type Conversion7 : DataTypeConversion  OutDataTypeStr=uint16
  Demux : Demux  Outputs=6
  Mux : Mux  Inputs=6
  Reshape{1..6} (6 alike) : Reshape  OutputDimensionality=Customize  OutputDimensions=[1,8]
  MSG1 : Outport
  MSG2 : Outport  Port=2
  MSG3 : Outport  Port=3
  MSG4 : Outport  Port=4
  MSG5 : Outport  Port=5
  MSG6 : Outport  Port=6
  wires:
  Data Store Read/1 -> Chart2/3(StartRobot)
  Current1/1 -> Mux/1
  Current2/1 -> Mux/2
  Current3/1 -> Mux/3
  Current4/1 -> Mux/4
  Current5/1 -> Mux/5
  Current6/1 -> Mux/6
  Mux/1 -> Data Type Conversion7/1
  Enable/1 -> Data Type Conversion1/1
  Data Type Conversion7/1 -> Chart2/1(Current)
  Demux/5 -> Reshape5/1
  Demux/4 -> Reshape4/1
  Demux/6 -> Reshape6/1
  Demux/3 -> Reshape3/1
  Demux/2 -> Reshape2/1
  Demux/1 -> Reshape1/1
  Data Type Conversion12/1 -> Demux/1
  Chart2/1(MSG) -> Data Type Conversion12/1
  Reshape1/1 -> MSG1/1
  Reshape2/1 -> MSG2/1
  Reshape3/1 -> MSG3/1
  Reshape4/1 -> MSG4/1
  Reshape5/1 -> MSG5/1
  Reshape6/1 -> MSG6/1
  Data Type Conversion1/1 -> Chart2/2(write)

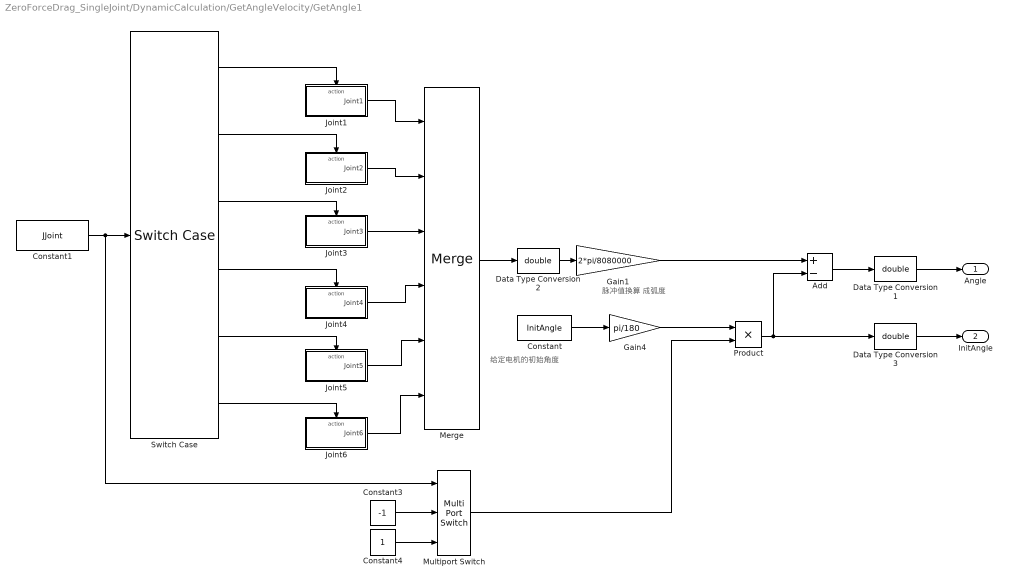
== system ZeroForceDrag_SingleJoint/DynamicCalculation/GetAngleVelocity/GetAngle1 ==
  note: 脉冲值换算
      | 成弧度
  note: 给定电机的初始角度
  Add : Sum  Inputs=+-
  Constant : Constant  Value=InitAngle
  Constant1 : Constant  Value=JJoint  OutDataTypeStr=uint8
  Constant3 : Constant  Value=-1
  Constant4 : Constant
  Data Type Conversion1 : DataTypeConversion  OutDataTypeStr=double
  Data Type Conversion2 : DataTypeConversion  OutDataTypeStr=double
  Data Type Conversion3 : DataTypeConversion  OutDataTypeStr=double
  Gain1 : Gain  Gain=2*pi/8080000
  Gain4 : Gain  Gain=pi/180
  Joint1 : Subsystem  TreatAsAtomicUnit=on
  Joint2 : Subsystem  TreatAsAtomicUnit=on
  Joint3 : Subsystem  TreatAsAtomicUnit=on
  Joint4 : Subsystem  TreatAsAtomicUnit=on
  Joint5 : Subsystem  TreatAsAtomicUnit=on
  Joint6 : Subsystem  TreatAsAtomicUnit=on
  Merge : Merge  Inputs=6  InitialOutput=0
  Multiport Switch : MultiPortSwitch  DataPortOrder=Specify indices  Inputs=2  DataPortIndices={3,[1,2,4,5,6]}
  Product : Product
  Switch Case : SwitchCase  CaseConditions={1 2 3 4 5 6}  ShowDefaultCase=off
  Angle : Outport
  InitAngle : Outport  Port=2
  wires:
  Data Type Conversion2/1 -> Gain1/1
  Data Type Conversion1/1 -> Angle/1
  Joint6/1(Joint6) -> Merge/6
  Joint5/1(Joint5) -> Merge/5
  Joint4/1(Joint4) -> Merge/4
  Joint3/1(Joint3) -> Merge/3
  Joint2/1(Joint2) -> Merge/2
  Joint1/1(Joint1) -> Merge/1
  Switch Case/6 -> Joint6/Action
  Switch Case/5 -> Joint5/Action
  Switch Case/4 -> Joint4/Action
  Switch Case/3 -> Joint3/Action
  Switch Case/2 -> Joint2/Action
  Switch Case/1 -> Joint1/Action
  Constant/1 -> Gain4/1
  Add/1 -> Data Type Conversion1/1
  Gain1/1 -> Add/1
  Gain4/1 -> Product/1
  Merge/1 -> Data Type Conversion2/1
  Multiport Switch/1 -> Product/2
  Constant4/1 -> Multiport Switch/3
  Constant3/1 -> Multiport Switch/2
  Constant1/1 -> Multiport Switch/1, Switch Case/1
  Product/1 -> Data Type Conversion3/1, Add/2
  Data Type Conversion3/1 -> InitAngle/1

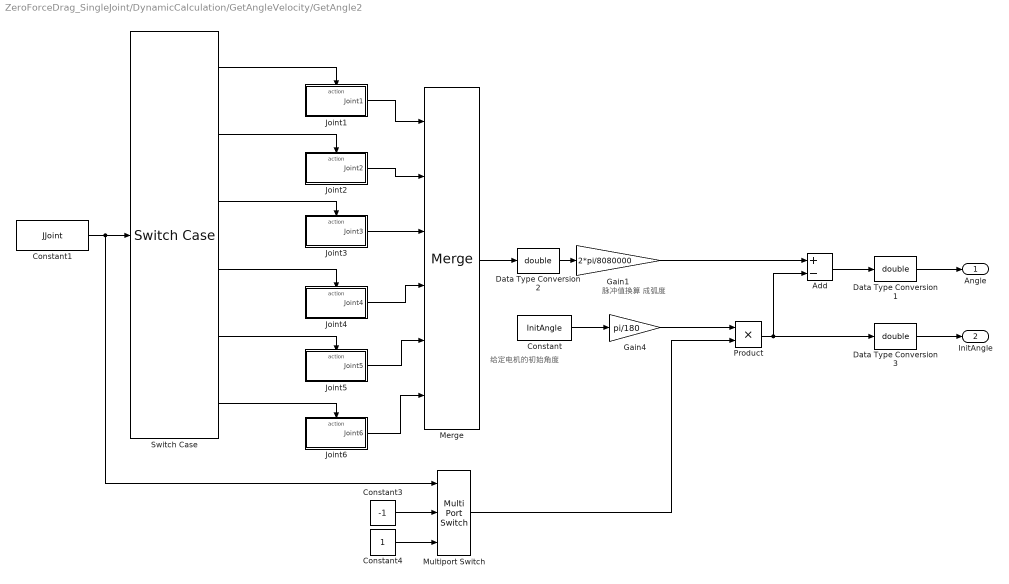
== system ZeroForceDrag_SingleJoint/DynamicCalculation/GetAngleVelocity/GetAngle2 ==
  note: 给定电机的初始角度
  note: 脉冲值换算
      | 成弧度
  Add : Sum  Inputs=+-
  Constant : Constant  Value=InitAngle
  Constant1 : Constant  Value=JJoint  OutDataTypeStr=uint8
  Constant3 : Constant  Value=-1
  Constant4 : Constant
  Data Type Conversion1 : DataTypeConversion  OutDataTypeStr=double
  Data Type Conversion2 : DataTypeConversion  OutDataTypeStr=double
  Data Type Conversion3 : DataTypeConversion  OutDataTypeStr=double
  Gain1 : Gain  Gain=2*pi/8080000
  Gain4 : Gain  Gain=pi/180
  Joint1 : Subsystem  TreatAsAtomicUnit=on
  Joint2 : Subsystem  TreatAsAtomicUnit=on
  Joint3 : Subsystem  TreatAsAtomicUnit=on
  Joint4 : Subsystem  TreatAsAtomicUnit=on
  Joint5 : Subsystem  TreatAsAtomicUnit=on
  Joint6 : Subsystem  TreatAsAtomicUnit=on
  Merge : Merge  Inputs=6  InitialOutput=0
  Multiport Switch : MultiPortSwitch  DataPortOrder=Specify indices  Inputs=2  DataPortIndices={3,[1,2,4,5,6]}
  Product : Product
  Switch Case : SwitchCase  CaseConditions={1 2 3 4 5 6}  ShowDefaultCase=off
  Angle : Outport
  InitAngle : Outport  Port=2
  wires:
  Data Type Conversion3/1 -> InitAngle/1
  Product/1 -> Add/2, Data Type Conversion3/1
  Constant1/1 -> Switch Case/1, Multiport Switch/1
  Constant3/1 -> Multiport Switch/2
  Constant4/1 -> Multiport Switch/3
  Multiport Switch/1 -> Product/2
  Merge/1 -> Data Type Conversion2/1
  Gain4/1 -> Product/1
  Gain1/1 -> Add/1
  Add/1 -> Data Type Conversion1/1
  Constant/1 -> Gain4/1
  Switch Case/1 -> Joint1/Action
  Switch Case/2 -> Joint2/Action
  Switch Case/3 -> Joint3/Action
  Switch Case/4 -> Joint4/Action
  Switch Case/5 -> Joint5/Action
  Switch Case/6 -> Joint6/Action
  Joint1/1(Joint1) -> Merge/1
  Joint2/1(Joint2) -> Merge/2
  Joint3/1(Joint3) -> Merge/3
  Joint4/1(Joint4) -> Merge/4
  Joint5/1(Joint5) -> Merge/5
  Joint6/1(Joint6) -> Merge/6
  Data Type Conversion1/1 -> Angle/1
  Data Type Conversion2/1 -> Gain1/1
